simulink model "DDCU_wxt_v02_forA"  (R2014a)
settings: Solver=FixedStepDiscrete  StartTime=0.0  StopTime=50  FixedStep=0.0005  RelTol=1e-3
InitFcn:
  | Veh_Par_wxt
values from neighbouring files (symbols this model uses):
  ag_thr = 0.4*g    (= 3.924)    [Veh_Par_wxt.m]
  B = 2.25    [Veh_Par_wxt.m]
  bra_pre_em = 12    [Veh_Par_wxt.m]
  bra_pre_gz2 = 12/3    (= 4)    [Veh_Par_wxt.m]
  bra_pre_gz34 = 12/3    (= 4)    [Veh_Par_wxt.m]
  bra_pre_yd = 12/2    (= 6)    [Veh_Par_wxt.m]
  brakepre_dem_data = [0 1 2 3 4 5 6 7 8 9 10 11 12]    [Veh_Par_wxt.m]
  brakeTrq_dem_data = [0 218.198 436.396 654.594 872.792 1090.99 1309.188 1527.386 1745.584 1963.782 2181.98 2400.178 2618.376]    [Veh_Par_wxt.m]
  bratrq_max = 4*2618.376    (= 10473.504)    [Veh_Par_wxt.m]
  eff_tran = 0.75    [Veh_Par_wxt.m]
  G = Mass*g    (= 36297)    [Veh_Par_wxt.m]
  kd1 = 1    [Veh_Par_wxt.m]
  kd2 = 1    [Veh_Par_wxt.m]
  kd3 = 1    [Veh_Par_wxt.m]
  ki1 = 1    [Veh_Par_wxt.m]
  ki2 = 1    [Veh_Par_wxt.m]
  ki3 = 1    [Veh_Par_wxt.m]
  kp1 = 1    [Veh_Par_wxt.m]
  kp2 = 1    [Veh_Par_wxt.m]
  kp3 = 1    [Veh_Par_wxt.m]
  L = 3.12    [Veh_Par_wxt.m]
  Radius = 0.20    (= 0.2)    [Veh_Par_wxt.m]
  s_opt_yi_add = 0.05    [Veh_Par_wxt.m]
  s_opt_zhuan_add = 0.05    [Veh_Par_wxt.m]
  spd_map_mot = [0 100 200 300 360 400 500 600 700 800 900]*tras_ratio    [Veh_Par_wxt.m]
  speed_thr_park = 5/3.6/Radius*30/pi    (= 66.3145596216)    [Veh_Par_wxt.m]
  trq_map_mot = [1200 1200 1200 1200 1200 1080 864 720 617 540 480]/tras_ratio    [Veh_Par_wxt.m]
  v_thr1_b = 5    [Veh_Par_wxt.m]
  v_thr2_b = 20    [Veh_Par_wxt.m]
  v_thr_park = 5    [Veh_Par_wxt.m]
undefined symbols (not defined in the file or in its folder): DiscIntNeverNeededParam
libraries: simulink x201, ec5744lib x19
(part 2 of 9)

== matlab function DDCU_wxt_v02_forA/MainControl/mode_control/center_steer/center_steer/容错控制/MATLAB Function ==
  data: trq_dem_l input; trq_dem_lf output; trq_dem_r input; trqlim_lf input; trqlim_lr input; trqlim_rf input; trqlim_rr input; guzhang_lf input; guzhang_lr input; guzhang_rf input; guzhang_rr input; trq_dem_lr output; trq_dem_rf output; trq_dem_rr output; bra_pre_l output; bra_pre_r output; bra_pre_yd input
function [trq_dem_lf,trq_dem_lr,trq_dem_rf,trq_dem_rr,bra_pre_l,bra_pre_r] = fcn(trq_dem_l,trq_dem_r,trqlim_lf,trqlim_lr,trqlim_rf,trqlim_rr,guzhang_lf,guzhang_lr,guzhang_rf,guzhang_rr,bra_pre_yd)
%#codegen
if guzhang_lf==0 && guzhang_lr==0 && guzhang_rf==0 && guzhang_rr==0    %0电机故障,平均分配
    trq_dem_lf=trq_dem_l/2;
    trq_dem_lr=trq_dem_l/2;
    trq_dem_rf=trq_dem_r/2;
    trq_dem_rr=trq_dem_r/2;
    bra_pre_l=0;
    bra_pre_r=0;
elseif  guzhang_lf==1 && guzhang_lr==0 && guzhang_rf==0 && guzhang_rr==0  %1电机故障，同侧电机进行力矩转移,跟行车不同，对侧不降扭。
    trq_dem_lf=0;
    trq_dem_lr=min(trq_dem_l,trqlim_lr);
    trq_dem_rf=trq_dem_r/2;
    trq_dem_rr=trq_dem_r/2;
    bra_pre_l=0;
    bra_pre_r=0;
elseif  guzhang_lf==0 && guzhang_lr==1 && guzhang_rf==0 && guzhang_rr==0
    trq_dem_lf=min(trq_dem_l,trqlim_lf);
    trq_dem_lr=0;
    trq_dem_rf=trq_dem_r/2;
    trq_dem_rr=trq_dem_r/2;
    bra_pre_l=0;
    bra_pre_r=0;
elseif  guzhang_lf==0 && guzhang_lr==0 && guzhang_rf==1 && guzhang_rr==0
    trq_dem_rf=0;
    trq_dem_rr=min(trq_dem_r,trqlim_rr);
    trq_dem_lf=trq_dem_l/2;
    trq_dem_lr=trq_dem_l/2;
    bra_pre_l=0;
    bra_pre_r=0;
elseif  guzhang_lf==0 && guzhang_lr==0 && guzhang_rf==0 && guzhang_rr==1
    trq_dem_rf=min(trq_dem_r,trqlim_rf);
    trq_dem_rr=0;
    trq_dem_lf=trq_dem_l/2;
    trq_dem_lr=trq_dem_l/2;
    bra_pre_l=0;
    bra_pre_r=0;
elseif  guzhang_lf==1 && guzhang_lr==1 && guzhang_rf==0 && guzhang_rr==0  %2电机故障，左侧双电机故障，左侧履带施加制动，改为原地转向
    trq_dem_lf=0;
    trq_dem_lr=0;
    trq_dem_rf=trq_dem_r/2;
    trq_dem_rr=trq_dem_r/2;
    bra_pre_l=bra_pre_yd;
    bra_pre_r=0;
elseif  guzhang_lf==0 && guzhang_lr==0 && guzhang_rf==1 && guzhang_rr==1  %右侧双电机故障
    trq_dem_lf=trq_dem_l/2;
    trq_dem_lr=trq_dem_l/2;
    trq_dem_rf=0;
    trq_dem_rr=0;
    bra_pre_l=0;
    bra_pre_r=bra_pre_yd;
    
elseif  guzhang_lf==1 && guzhang_lr==0 && guzhang_rf==1 && guzhang_rr==0 %2电机故障，对侧双电机故障,有4种情况,前两电机故障
    trq_dem_lf=0;
    trq_dem_rf=0;
    trq_dem_lr=min(trq_dem_l,trqlim_lr);
    trq_dem_rr=min(trq_dem_r,trqlim_rr);
    bra_pre_l=0;
    bra_pre_r=0;
elseif  guzhang_lf==0 && guzhang_lr==1 && guzhang_rf==0 && guzhang_rr==0 %后两电机故障
    trq_dem_lr=0;
    trq_dem_rr=0;
    trq_dem_lf=min(trq_dem_l,trqlim_lf);
    trq_dem_rf=min(trq_dem_r,trqlim_rf);
    bra_pre_l=0;
    bra_pre_r=0;
elseif  guzhang_lf==0 && guzhang_lr==1 && guzhang_rf==0 && guzhang_rr==0 %左前电机和右后电机故障
    trq_dem_lf=0;
    trq_dem_rr=0;
    trq_dem_lr=min(trq_dem_l,trqlim_lr);
    trq_dem_rf=min(trq_dem_r,trqlim_rf);
    bra_pre_l=0;
    bra_pre_r=0;
elseif  guzhang_lf==0 && guzhang_lr==1 && guzhang_rf==0 && guzhang_rr==0 %左后电机和右前电机故障
    trq_dem_lr=0;
    trq_dem_rf=0;
    trq_dem_lf=min(trq_dem_l,trqlim_lf);
    trq_dem_rr=min(trq_dem_r,trqlim_rr);
    bra_pre_l=0;
    bra_pre_r=0;
elseif guzhang_lf==1 && guzhang_lr==1 && guzhang_rf==1 && guzhang_rr==0   % 三电机故障
    trq_dem_lf=0;
    trq_dem_lr=0;
    trq_dem_rf=0;
    trq_dem_rr=min(trq_dem_r,trqlim_rr);
    bra_pre_l=bra_pre_yd;
    bra_pre_r=0;
elseif guzhang_lf==1 && guzhang_lr==1 && guzhang_rf==0 && guzhang_rr==1
    trq_dem_lf=0;
    trq_dem_lr=0;
    trq_dem_rf=min(trq_dem_r,trqlim_rf);
    trq_dem_rr=0;
    bra_pre_l=bra_pre_yd;
    bra_pre_r=0;
elseif guzhang_lf==1 && guzhang_lr==0 && guzhang_rf==1 && guzhang_rr==1
    trq_dem_lf=0;
    trq_dem_lr=min(trq_dem_l,trqlim_lr);
    trq_dem_rf=0;
    trq_dem_rr=0;
    bra_pre_l=0;
    bra_pre_r=bra_pre_yd;
elseif guzhang_lf==0 && guzhang_lr==1 && guzhang_rf==1 && guzhang_rr==1
    trq_dem_lf=min(trq_dem_l,trqlim_lf);
    trq_dem_lr=0;
    trq_dem_rf=0;
    trq_dem_rr=0;
    bra_pre_l=0;
    bra_pre_r=bra_pre_yd;
else
    %     guzhang_lf==1 && guzhang_lr==1 && guzhang_rf==1 && guzhang_rr==1 %四电机故障
    trq_dem_lf=0;
    trq_dem_lr=0;
    trq_dem_rf=0;
    trq_dem_rr=0;
    bra_pre_l=0;
    bra_pre_r=0;
end
end

== system DDCU_wxt_v02_forA/OutputSignalProcess/VCU_MCU2_replace ==
  M4SpeedSet_in : Inport
  M3SpeedSet_in : Inport  Port=2
  MCU2HeartBeat_in : Inport  Port=3
  M4SpeedLimit_in : Inport  Port=4
  M4Mode_in : Inport  Port=5
  M4Enable_in : Inport  Port=6
  M4Drive_in : Inport  Port=7
  M3SpeedLimit_in : Inport  Port=8
  M3Mode_in : Inport  Port=9
  M3Enable_in : Inport  Port=10
  M3Drive_in : Inport  Port=11
  Conv{1..8} (8 alike) : DataTypeConversion
  M3Drive : Subsystem
  M3Enable : Subsystem
  M3Mode : Subsystem
  M3SpeedLimit : Subsystem
  M3SpeedSet : Subsystem
  M4Drive : Subsystem
  M4Enable : Subsystem
  M4Mode : Subsystem
  M4SpeedLimit : Subsystem
  M4SpeedSet : Subsystem
  MCU2HeartBeat : Subsystem
  VCU_MCU2_replace_DLC : Constant  Value=8  OutDataTypeStr=uint8
  VCU_MCU2_replace_DLC_Out : Terminator
  VCU_MCU2_replace_ID : Constant  Value=2348937234  OutDataTypeStr=single
  VCU_MCU2_replace_ID_Out : Terminator
  VCU_MCU2_replace_mux : Mux  Inputs=8
  or{1..8} (8 alike) : simulink/Logic and Bit Operations/Bitwise Operator  logicop=OR  UseBitMask=off  NumInputPorts=11  BitMask=bin2dec('11011001')  BitMaskRealWorld=Stored Integer
  output : Outport
  wires:
  VCU_MCU2_replace_mux/1 -> output/1
  M4SpeedSet/1(output1) -> or1/1
  M4SpeedSet/2(output2) -> or2/1
  M4SpeedSet/3(output3) -> or3/1
  M4SpeedSet/4(output4) -> or4/1
  M4SpeedSet/5(output5) -> or5/1
  M4SpeedSet/6(output6) -> or6/1
  M4SpeedSet/7(output7) -> or7/1
  M4SpeedSet/8(output8) -> or8/1
  M3SpeedSet/1(output1) -> or1/2
  M3SpeedSet/2(output2) -> or2/2
  M3SpeedSet/3(output3) -> or3/2
  M3SpeedSet/4(output4) -> or4/2
  M3SpeedSet/5(output5) -> or5/2
  M3SpeedSet/6(output6) -> or6/2
  M3SpeedSet/7(output7) -> or7/2
  M3SpeedSet/8(output8) -> or8/2
  MCU2HeartBeat/1(output1) -> or1/3
  MCU2HeartBeat/2(output2) -> or2/3
  MCU2HeartBeat/3(output3) -> or3/3
  MCU2HeartBeat/4(output4) -> or4/3
  MCU2HeartBeat/5(output5) -> or5/3
  MCU2HeartBeat/6(output6) -> or6/3
  MCU2HeartBeat/7(output7) -> or7/3
  MCU2HeartBeat/8(output8) -> or8/3
  M4SpeedLimit/1(output1) -> or1/4
  M4SpeedLimit/2(output2) -> or2/4
  M4SpeedLimit/3(output3) -> or3/4
  M4SpeedLimit/4(output4) -> or4/4
  M4SpeedLimit/5(output5) -> or5/4
  M4SpeedLimit/6(output6) -> or6/4
  M4SpeedLimit/7(output7) -> or7/4
  M4SpeedLimit/8(output8) -> or8/4
  M4Mode/1(output1) -> or1/5
  M4Mode/2(output2) -> or2/5
  M4Mode/3(output3) -> or3/5
  M4Mode/4(output4) -> or4/5
  M4Mode/5(output5) -> or5/5
  M4Mode/6(output6) -> or6/5
  M4Mode/7(output7) -> or7/5
  M4Mode/8(output8) -> or8/5
  M4Enable/1(output1) -> or1/6
  M4Enable/2(output2) -> or2/6
  M4Enable/3(output3) -> or3/6
  M4Enable/4(output4) -> or4/6
  M4Enable/5(output5) -> or5/6
  M4Enable/6(output6) -> or6/6
  M4Enable/7(output7) -> or7/6
  M4Enable/8(output8) -> or8/6
  M4Drive/1(output1) -> or1/7
  M4Drive/2(output2) -> or2/7
  M4Drive/3(output3) -> or3/7
  M4Drive/4(output4) -> or4/7
  M4Drive/5(output5) -> or5/7
  M4Drive/6(output6) -> or6/7
  M4Drive/7(output7) -> or7/7
  M4Drive/8(output8) -> or8/7
  M3SpeedLimit/1(output1) -> or1/8
  M3SpeedLimit/2(output2) -> or2/8
  M3SpeedLimit/3(output3) -> or3/8
  M3SpeedLimit/4(output4) -> or4/8
  M3SpeedLimit/5(output5) -> or5/8
  M3SpeedLimit/6(output6) -> or6/8
  M3SpeedLimit/7(output7) -> or7/8
  M3SpeedLimit/8(output8) -> or8/8
  M3Mode/1(output1) -> or1/9
  M3Mode/2(output2) -> or2/9
  M3Mode/3(output3) -> or3/9
  M3Mode/4(output4) -> or4/9
  M3Mode/5(output5) -> or5/9
  M3Mode/6(output6) -> or6/9
  M3Mode/7(output7) -> or7/9
  M3Mode/8(output8) -> or8/9
  M3Enable/1(output1) -> or1/10
  M3Enable/2(output2) -> or2/10
  M3Enable/3(output3) -> or3/10
  M3Enable/4(output4) -> or4/10
  M3Enable/5(output5) -> or5/10
  M3Enable/6(output6) -> or6/10
  M3Enable/7(output7) -> or7/10
  M3Enable/8(output8) -> or8/10
  M3Drive/1(output1) -> or1/11
  M3Drive/2(output2) -> or2/11
  M3Drive/3(output3) -> or3/11
  M3Drive/4(output4) -> or4/11
  M3Drive/5(output5) -> or5/11
  M3Drive/6(output6) -> or6/11
  M3Drive/7(output7) -> or7/11
  M3Drive/8(output8) -> or8/11
  or1/1 -> Conv1/1
  Conv1/1 -> VCU_MCU2_replace_mux/1
  or2/1 -> Conv2/1
  Conv2/1 -> VCU_MCU2_replace_mux/2
  or3/1 -> Conv3/1
  Conv3/1 -> VCU_MCU2_replace_mux/3
  or4/1 -> Conv4/1
  Conv4/1 -> VCU_MCU2_replace_mux/4
  or5/1 -> Conv5/1
  Conv5/1 -> VCU_MCU2_replace_mux/5
  or6/1 -> Conv6/1
  Conv6/1 -> VCU_MCU2_replace_mux/6
  or7/1 -> Conv7/1
  Conv7/1 -> VCU_MCU2_replace_mux/7
  or8/1 -> Conv8/1
  Conv8/1 -> VCU_MCU2_replace_mux/8
  VCU_MCU2_replace_ID/1 -> VCU_MCU2_replace_ID_Out/1
  VCU_MCU2_replace_DLC/1 -> VCU_MCU2_replace_DLC_Out/1
  M4SpeedSet_in/1 -> M4SpeedSet/1(M4SpeedSet)
  M3SpeedSet_in/1 -> M3SpeedSet/1(M3SpeedSet)
  MCU2HeartBeat_in/1 -> MCU2HeartBeat/1(MCU2HeartBeat)
  M4SpeedLimit_in/1 -> M4SpeedLimit/1(M4SpeedLimit)
  M4Mode_in/1 -> M4Mode/1(M4Mode)
  M4Enable_in/1 -> M4Enable/1(M4Enable)
  M4Drive_in/1 -> M4Drive/1(M4Drive)
  M3SpeedLimit_in/1 -> M3SpeedLimit/1(M3SpeedLimit)
  M3Mode_in/1 -> M3Mode/1(M3Mode)
  M3Enable_in/1 -> M3Enable/1(M3Enable)
  M3Drive_in/1 -> M3Drive/1(M3Drive)

== system DDCU_wxt_v02_forA/OutputSignalProcess/VCU_Park ==
  ParkEnable_in : Inport
  Conv{1..8} (8 alike) : DataTypeConversion
  ParkEnable : Subsystem
  VCU_Park_DLC : Constant  Value=8  OutDataTypeStr=uint8
  VCU_Park_DLC_Out : Terminator
  VCU_Park_ID : Constant  Value=2281988666  OutDataTypeStr=single
  VCU_Park_ID_Out : Terminator
  VCU_Park_mux : Mux  Inputs=8
  or{1..8} (8 alike) : simulink/Logic and Bit Operations/Bitwise Operator  logicop=OR  UseBitMask=off  BitMask=bin2dec('11011001')  BitMaskRealWorld=Stored Integer
  output : Outport
  wires:
  VCU_Park_mux/1 -> output/1
  ParkEnable/1(output1) -> or1/1
  ParkEnable/2(output2) -> or2/1
  ParkEnable/3(output3) -> or3/1
  ParkEnable/4(output4) -> or4/1
  ParkEnable/5(output5) -> or5/1
  ParkEnable/6(output6) -> or6/1
  ParkEnable/7(output7) -> or7/1
  ParkEnable/8(output8) -> or8/1
  or1/1 -> Conv1/1
  Conv1/1 -> VCU_Park_mux/1
  or2/1 -> Conv2/1
  Conv2/1 -> VCU_Park_mux/2
  or3/1 -> Conv3/1
  Conv3/1 -> VCU_Park_mux/3
  or4/1 -> Conv4/1
  Conv4/1 -> VCU_Park_mux/4
  or5/1 -> Conv5/1
  Conv5/1 -> VCU_Park_mux/5
  or6/1 -> Conv6/1
  Conv6/1 -> VCU_Park_mux/6
  or7/1 -> Conv7/1
  Conv7/1 -> VCU_Park_mux/7
  or8/1 -> Conv8/1
  Conv8/1 -> VCU_Park_mux/8
  VCU_Park_ID/1 -> VCU_Park_ID_Out/1
  VCU_Park_DLC/1 -> VCU_Park_DLC_Out/1
  ParkEnable_in/1 -> ParkEnable/1(ParkEnable)

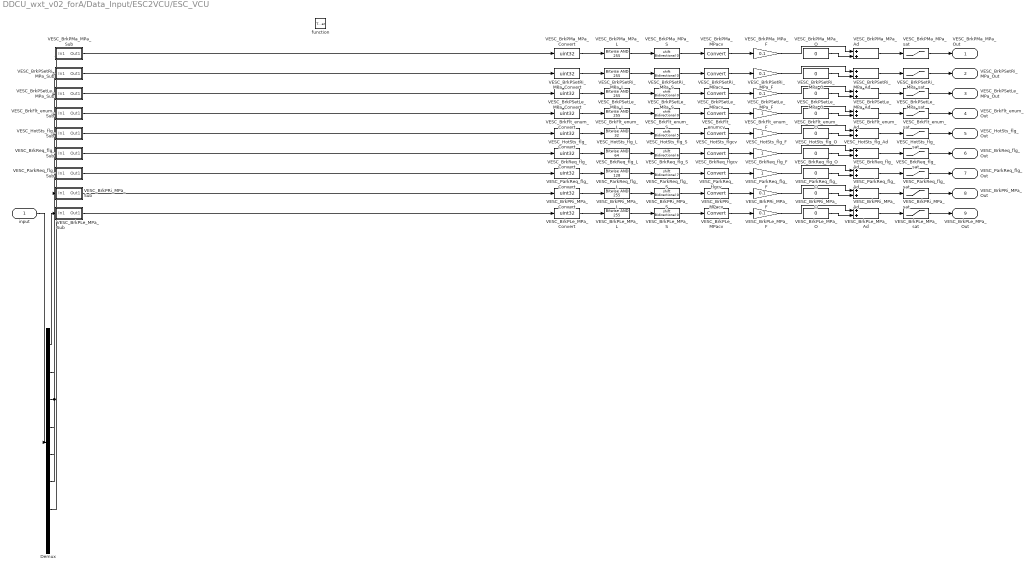
== system DDCU_wxt_v02_forA/Data_Input/ESC2VCU/ESC_VCU ==
  input : Inport
  function : TriggerPort  TriggerType=function-call
  Demux : Demux  Outputs=8
  VESC_BrkFlt_enum_Ad : Sum
  VESC_BrkFlt_enum_Convert : DataTypeConversion  OutDataTypeStr=uint32
  VESC_BrkFlt_enum_F : Gain
  VESC_BrkFlt_enum_L : simulink/Logic and Bit Operations/Bitwise Operator  logicop=AND  UseBitMask=on  BitMask=255  BitMaskRealWorld=Stored Integer
  VESC_BrkFlt_enum_O : Constant  Value=0  OutDataTypeStr=single
  VESC_BrkFlt_enum_S : ArithShift
  VESC_BrkFlt_enum_Sub : Subsystem
  VESC_BrkFlt_enum_sat : Saturate  UpperLimit=255  LowerLimit=0
  VESC_BrkFlt_enumcv : DataTypeConversion
  VESC_BrkPLe_MPa_Ad : Sum
  VESC_BrkPLe_MPa_Convert : DataTypeConversion  OutDataTypeStr=uint32
  VESC_BrkPLe_MPa_F : Gain  Gain=0.1
  VESC_BrkPLe_MPa_L : simulink/Logic and Bit Operations/Bitwise Operator  logicop=AND  UseBitMask=on  BitMask=255  BitMaskRealWorld=Stored Integer
  VESC_BrkPLe_MPa_O : Constant  Value=0  OutDataTypeStr=single
  VESC_BrkPLe_MPa_S : ArithShift
  VESC_BrkPLe_MPa_Sub : Subsystem
  VESC_BrkPLe_MPa_sat : Saturate  UpperLimit=25.5  LowerLimit=0
  VESC_BrkPLe_MPacv : DataTypeConversion
  VESC_BrkPMa_MPa_Ad : Sum
  VESC_BrkPMa_MPa_Convert : DataTypeConversion  OutDataTypeStr=uint32
  VESC_BrkPMa_MPa_F : Gain  Gain=0.1
  VESC_BrkPMa_MPa_L : simulink/Logic and Bit Operations/Bitwise Operator  logicop=AND  UseBitMask=on  BitMask=255  BitMaskRealWorld=Stored Integer
  VESC_BrkPMa_MPa_O : Constant  Value=0  OutDataTypeStr=single
  VESC_BrkPMa_MPa_S : ArithShift
  VESC_BrkPMa_MPa_Sub : Subsystem
  VESC_BrkPMa_MPa_sat : Saturate  UpperLimit=25.5  LowerLimit=0
  VESC_BrkPMa_MPacv : DataTypeConversion
  VESC_BrkPRi_MPa_Ad : Sum
  VESC_BrkPRi_MPa_Convert : DataTypeConversion  OutDataTypeStr=uint32
  VESC_BrkPRi_MPa_F : Gain  Gain=0.1
  VESC_BrkPRi_MPa_L : simulink/Logic and Bit Operations/Bitwise Operator  logicop=AND  UseBitMask=on  BitMask=255  BitMaskRealWorld=Stored Integer
  VESC_BrkPRi_MPa_O : Constant  Value=0  OutDataTypeStr=single
  VESC_BrkPRi_MPa_S : ArithShift
  VESC_BrkPRi_MPa_Sub : Subsystem
  VESC_BrkPRi_MPa_sat : Saturate  UpperLimit=25.5  LowerLimit=0
  VESC_BrkPRi_MPacv : DataTypeConversion
  VESC_BrkPSetLe_MPa_Ad : Sum
  VESC_BrkPSetLe_MPa_Convert : DataTypeConversion  OutDataTypeStr=uint32
  VESC_BrkPSetLe_MPa_F : Gain  Gain=0.1
  VESC_BrkPSetLe_MPa_L : simulink/Logic and Bit Operations/Bitwise Operator  logicop=AND  UseBitMask=on  BitMask=255  BitMaskRealWorld=Stored Integer
  VESC_BrkPSetLe_MPa_O : Constant  Value=0  OutDataTypeStr=single
  VESC_BrkPSetLe_MPa_S : ArithShift
  VESC_BrkPSetLe_MPa_Sub : Subsystem
  VESC_BrkPSetLe_MPa_sat : Saturate  UpperLimit=25.5  LowerLimit=0
  VESC_BrkPSetLe_MPacv : DataTypeConversion
  VESC_BrkPSetRi_MPa_Ad : Sum
  VESC_BrkPSetRi_MPa_Convert : DataTypeConversion  OutDataTypeStr=uint32
  VESC_BrkPSetRi_MPa_F : Gain  Gain=0.1
  VESC_BrkPSetRi_MPa_L : simulink/Logic and Bit Operations/Bitwise Operator  logicop=AND  UseBitMask=on  BitMask=255  BitMaskRealWorld=Stored Integer
  VESC_BrkPSetRi_MPa_O : Constant  Value=0  OutDataTypeStr=single
  VESC_BrkPSetRi_MPa_S : ArithShift
  VESC_BrkPSetRi_MPa_Sub : Subsystem
  VESC_BrkPSetRi_MPa_sat : Saturate  UpperLimit=25.5  LowerLimit=0
  VESC_BrkPSetRi_MPacv : DataTypeConversion
  VESC_BrkReq_flg_Ad : Sum
  VESC_BrkReq_flg_Convert : DataTypeConversion  OutDataTypeStr=uint32
  VESC_BrkReq_flg_F : Gain
  VESC_BrkReq_flg_L : simulink/Logic and Bit Operations/Bitwise Operator  logicop=AND  UseBitMask=on  BitMask=64  BitMaskRealWorld=Stored Integer
  VESC_BrkReq_flg_O : Constant  Value=0  OutDataTypeStr=single
  VESC_BrkReq_flg_S : ArithShift  BitShiftNumber=6
  VESC_BrkReq_flg_Sub : Subsystem
  VESC_BrkReq_flg_sat : Saturate  UpperLimit=1  LowerLimit=0
  VESC_BrkReq_flgcv : DataTypeConversion
  VESC_HotSts_flg_Ad : Sum
  VESC_HotSts_flg_Convert : DataTypeConversion  OutDataTypeStr=uint32
  VESC_HotSts_flg_F : Gain
  VESC_HotSts_flg_L : simulink/Logic and Bit Operations/Bitwise Operator  logicop=AND  UseBitMask=on  BitMask=32  BitMaskRealWorld=Stored Integer
  VESC_HotSts_flg_O : Constant  Value=0  OutDataTypeStr=single
  VESC_HotSts_flg_S : ArithShift  BitShiftNumber=5
  VESC_HotSts_flg_Sub : Subsystem
  VESC_HotSts_flg_sat : Saturate  UpperLimit=1  LowerLimit=0
  VESC_HotSts_flgcv : DataTypeConversion
  VESC_ParkReq_flg_Ad : Sum
  VESC_ParkReq_flg_Convert : DataTypeConversion  OutDataTypeStr=uint32
  VESC_ParkReq_flg_F : Gain
  VESC_ParkReq_flg_L : simulink/Logic and Bit Operations/Bitwise Operator  logicop=AND  UseBitMask=on  BitMask=128  BitMaskRealWorld=Stored Integer
  VESC_ParkReq_flg_O : Constant  Value=0  OutDataTypeStr=single
  VESC_ParkReq_flg_S : ArithShift  BitShiftNumber=7
  VESC_ParkReq_flg_Sub : Subsystem
  VESC_ParkReq_flg_sat : Saturate  UpperLimit=1  LowerLimit=0
  VESC_ParkReq_flgcv : DataTypeConversion
  VESC_BrkPMa_MPa_Out : Outport
  VESC_BrkPSetRi_MPa_Out : Outport  Port=2
  VESC_BrkPSetLe_MPa_Out : Outport  Port=3
  VESC_BrkFlt_enum_Out : Outport  Port=4
  VESC_HotSts_flg_Out : Outport  Port=5
  VESC_BrkReq_flg_Out : Outport  Port=6
  VESC_ParkReq_flg_Out : Outport  Port=7
  VESC_BrkPRi_MPa_Out : Outport  Port=8
  VESC_BrkPLe_MPa_Out : Outport  Port=9
  wires:
  VESC_BrkPMa_MPa_F/1 -> VESC_BrkPMa_MPa_Ad/1
  VESC_BrkPMa_MPa_O/1 -> VESC_BrkPMa_MPa_Ad/2
  VESC_BrkPMa_MPa_Ad/1 -> VESC_BrkPMa_MPa_sat/1
  VESC_BrkPMa_MPa_sat/1 -> VESC_BrkPMa_MPa_Out/1
  Demux/7 -> VESC_BrkPMa_MPa_Sub/1(In1)
  VESC_BrkPMa_MPa_Sub/1(Out1) -> VESC_BrkPMa_MPa_Convert/1
  VESC_BrkPMa_MPa_Convert/1 -> VESC_BrkPMa_MPa_L/1
  VESC_BrkPMa_MPa_L/1 -> VESC_BrkPMa_MPa_S/1
  VESC_BrkPMa_MPa_S/1 -> VESC_BrkPMa_MPacv/1
  VESC_BrkPMa_MPacv/1 -> VESC_BrkPMa_MPa_F/1
  VESC_BrkPSetRi_MPa_F/1 -> VESC_BrkPSetRi_MPa_Ad/1
  VESC_BrkPSetRi_MPa_O/1 -> VESC_BrkPSetRi_MPa_Ad/2
  VESC_BrkPSetRi_MPa_Ad/1 -> VESC_BrkPSetRi_MPa_sat/1
  VESC_BrkPSetRi_MPa_sat/1 -> VESC_BrkPSetRi_MPa_Out/1
  Demux/6 -> VESC_BrkPSetRi_MPa_Sub/1(In1)
  VESC_BrkPSetRi_MPa_Sub/1(Out1) -> VESC_BrkPSetRi_MPa_Convert/1
  VESC_BrkPSetRi_MPa_Convert/1 -> VESC_BrkPSetRi_MPa_L/1
  VESC_BrkPSetRi_MPa_L/1 -> VESC_BrkPSetRi_MPa_S/1
  VESC_BrkPSetRi_MPa_S/1 -> VESC_BrkPSetRi_MPacv/1
  VESC_BrkPSetRi_MPacv/1 -> VESC_BrkPSetRi_MPa_F/1
  VESC_BrkPSetLe_MPa_F/1 -> VESC_BrkPSetLe_MPa_Ad/1
  VESC_BrkPSetLe_MPa_O/1 -> VESC_BrkPSetLe_MPa_Ad/2
  VESC_BrkPSetLe_MPa_Ad/1 -> VESC_BrkPSetLe_MPa_sat/1
  VESC_BrkPSetLe_MPa_sat/1 -> VESC_BrkPSetLe_MPa_Out/1
  Demux/5 -> VESC_BrkPSetLe_MPa_Sub/1(In1)
  VESC_BrkPSetLe_MPa_Sub/1(Out1) -> VESC_BrkPSetLe_MPa_Convert/1
  VESC_BrkPSetLe_MPa_Convert/1 -> VESC_BrkPSetLe_MPa_L/1
  VESC_BrkPSetLe_MPa_L/1 -> VESC_BrkPSetLe_MPa_S/1
  VESC_BrkPSetLe_MPa_S/1 -> VESC_BrkPSetLe_MPacv/1
  VESC_BrkPSetLe_MPacv/1 -> VESC_BrkPSetLe_MPa_F/1
  VESC_BrkFlt_enum_F/1 -> VESC_BrkFlt_enum_Ad/1
  VESC_BrkFlt_enum_O/1 -> VESC_BrkFlt_enum_Ad/2
  VESC_BrkFlt_enum_Ad/1 -> VESC_BrkFlt_enum_sat/1
  VESC_BrkFlt_enum_sat/1 -> VESC_BrkFlt_enum_Out/1
  Demux/4 -> VESC_BrkFlt_enum_Sub/1(In1)
  VESC_BrkFlt_enum_Sub/1(Out1) -> VESC_BrkFlt_enum_Convert/1
  VESC_BrkFlt_enum_Convert/1 -> VESC_BrkFlt_enum_L/1
  VESC_BrkFlt_enum_L/1 -> VESC_BrkFlt_enum_S/1
  VESC_BrkFlt_enum_S/1 -> VESC_BrkFlt_enumcv/1
  VESC_BrkFlt_enumcv/1 -> VESC_BrkFlt_enum_F/1
  VESC_HotSts_flg_F/1 -> VESC_HotSts_flg_Ad/1
  VESC_HotSts_flg_O/1 -> VESC_HotSts_flg_Ad/2
  VESC_HotSts_flg_Ad/1 -> VESC_HotSts_flg_sat/1
  VESC_HotSts_flg_sat/1 -> VESC_HotSts_flg_Out/1
  Demux/3 -> VESC_BrkReq_flg_Sub/1(In1), VESC_ParkReq_flg_Sub/1(In1), VESC_HotSts_flg_Sub/1(In1)
  VESC_HotSts_flg_Sub/1(Out1) -> VESC_HotSts_flg_Convert/1
  VESC_HotSts_flg_Convert/1 -> VESC_HotSts_flg_L/1
  VESC_HotSts_flg_L/1 -> VESC_HotSts_flg_S/1
  VESC_HotSts_flg_S/1 -> VESC_HotSts_flgcv/1
  VESC_HotSts_flgcv/1 -> VESC_HotSts_flg_F/1
  VESC_BrkReq_flg_F/1 -> VESC_BrkReq_flg_Ad/1
  VESC_BrkReq_flg_O/1 -> VESC_BrkReq_flg_Ad/2
  VESC_BrkReq_flg_Ad/1 -> VESC_BrkReq_flg_sat/1
  VESC_BrkReq_flg_sat/1 -> VESC_BrkReq_flg_Out/1
  VESC_BrkReq_flg_Sub/1(Out1) -> VESC_BrkReq_flg_Convert/1
  VESC_BrkReq_flg_Convert/1 -> VESC_BrkReq_flg_L/1
  VESC_BrkReq_flg_L/1 -> VESC_BrkReq_flg_S/1
  VESC_BrkReq_flg_S/1 -> VESC_BrkReq_flgcv/1
  VESC_BrkReq_flgcv/1 -> VESC_BrkReq_flg_F/1
  VESC_ParkReq_flg_F/1 -> VESC_ParkReq_flg_Ad/1
  VESC_ParkReq_flg_O/1 -> VESC_ParkReq_flg_Ad/2
  VESC_ParkReq_flg_Ad/1 -> VESC_ParkReq_flg_sat/1
  VESC_ParkReq_flg_sat/1 -> VESC_ParkReq_flg_Out/1
  VESC_ParkReq_flg_Sub/1(Out1) -> VESC_ParkReq_flg_Convert/1
  VESC_ParkReq_flg_Convert/1 -> VESC_ParkReq_flg_L/1
  VESC_ParkReq_flg_L/1 -> VESC_ParkReq_flg_S/1
  VESC_ParkReq_flg_S/1 -> VESC_ParkReq_flgcv/1
  VESC_ParkReq_flgcv/1 -> VESC_ParkReq_flg_F/1
  VESC_BrkPRi_MPa_F/1 -> VESC_BrkPRi_MPa_Ad/1
  VESC_BrkPRi_MPa_O/1 -> VESC_BrkPRi_MPa_Ad/2
  VESC_BrkPRi_MPa_Ad/1 -> VESC_BrkPRi_MPa_sat/1
  VESC_BrkPRi_MPa_sat/1 -> VESC_BrkPRi_MPa_Out/1
  Demux/2 -> VESC_BrkPRi_MPa_Sub/1(In1)
  VESC_BrkPRi_MPa_Sub/1(Out1) -> VESC_BrkPRi_MPa_Convert/1
  VESC_BrkPRi_MPa_Convert/1 -> VESC_BrkPRi_MPa_L/1
  VESC_BrkPRi_MPa_L/1 -> VESC_BrkPRi_MPa_S/1
  VESC_BrkPRi_MPa_S/1 -> VESC_BrkPRi_MPacv/1
  VESC_BrkPRi_MPacv/1 -> VESC_BrkPRi_MPa_F/1
  VESC_BrkPLe_MPa_F/1 -> VESC_BrkPLe_MPa_Ad/1
  VESC_BrkPLe_MPa_O/1 -> VESC_BrkPLe_MPa_Ad/2
  VESC_BrkPLe_MPa_Ad/1 -> VESC_BrkPLe_MPa_sat/1
  VESC_BrkPLe_MPa_sat/1 -> VESC_BrkPLe_MPa_Out/1
  Demux/1 -> VESC_BrkPLe_MPa_Sub/1(In1)
  VESC_BrkPLe_MPa_Sub/1(Out1) -> VESC_BrkPLe_MPa_Convert/1
  VESC_BrkPLe_MPa_Convert/1 -> VESC_BrkPLe_MPa_L/1
  VESC_BrkPLe_MPa_L/1 -> VESC_BrkPLe_MPa_S/1
  VESC_BrkPLe_MPa_S/1 -> VESC_BrkPLe_MPacv/1
  VESC_BrkPLe_MPacv/1 -> VESC_BrkPLe_MPa_F/1
  input/1 -> Demux/1

== system DDCU_wxt_v02_forA/Data_Input/ESC2VCU/Park1_VCU ==
  input : Inport
  function : TriggerPort  TriggerType=function-call
  Demux : Demux  Outputs=8
  ParkZiJian_Ad : Sum
  ParkZiJian_Convert : DataTypeConversion  OutDataTypeStr=uint32
  ParkZiJian_F : Gain
  ParkZiJian_L : simulink/Logic and Bit Operations/Bitwise Operator  logicop=AND  UseBitMask=on  BitMask=1  BitMaskRealWorld=Stored Integer
  ParkZiJian_O : Constant  Value=0  OutDataTypeStr=single
  ParkZiJian_S : ArithShift
  ParkZiJian_Sub : Subsystem
  ParkZiJian_sat : Saturate  UpperLimit=1  LowerLimit=0
  ParkZiJiancv : DataTypeConversion
  ParkZiJian_Out : Outport
  wires:
  ParkZiJian_F/1 -> ParkZiJian_Ad/1
  ParkZiJian_O/1 -> ParkZiJian_Ad/2
  ParkZiJian_Ad/1 -> ParkZiJian_sat/1
  ParkZiJian_sat/1 -> ParkZiJian_Out/1
  Demux/2 -> ParkZiJian_Sub/1(In1)
  ParkZiJian_Sub/1(Out1) -> ParkZiJian_Convert/1
  ParkZiJian_Convert/1 -> ParkZiJian_L/1
  ParkZiJian_L/1 -> ParkZiJian_S/1
  ParkZiJian_S/1 -> ParkZiJiancv/1
  ParkZiJiancv/1 -> ParkZiJian_F/1
  input/1 -> Demux/1

== system DDCU_wxt_v02_forA/Data_Input/ESC2VCU/Park2_VCU ==
  input : Inport
  function : TriggerPort  TriggerType=function-call
  Demux : Demux  Outputs=8
  ParkState_Ad : Sum
  ParkState_Convert : DataTypeConversion  OutDataTypeStr=uint32
  ParkState_F : Gain
  ParkState_L : simulink/Logic and Bit Operations/Bitwise Operator  logicop=AND  UseBitMask=on  BitMask=1  BitMaskRealWorld=Stored Integer
  ParkState_O : Constant  Value=0  OutDataTypeStr=single
  ParkState_S : ArithShift
  ParkState_Sub : Subsystem
  ParkState_sat : Saturate  UpperLimit=1  LowerLimit=0
  ParkStatecv : DataTypeConversion
  ParkState_Out : Outport
  wires:
  ParkState_F/1 -> ParkState_Ad/1
  ParkState_O/1 -> ParkState_Ad/2
  ParkState_Ad/1 -> ParkState_sat/1
  ParkState_sat/1 -> ParkState_Out/1
  Demux/2 -> ParkState_Sub/1(In1)
  ParkState_Sub/1(Out1) -> ParkState_Convert/1
  ParkState_Convert/1 -> ParkState_L/1
  ParkState_L/1 -> ParkState_S/1
  ParkState_S/1 -> ParkStatecv/1
  ParkStatecv/1 -> ParkState_F/1
  input/1 -> Demux/1

== system DDCU_wxt_v02_forA/Data_Input/HCU2VCU/HCU1_VCU ==
  input : Inport
  function : TriggerPort  TriggerType=function-call
  Demux : Demux  Outputs=8
  HCUState_Ad : Sum
  HCUState_Convert : DataTypeConversion  OutDataTypeStr=uint32
  HCUState_F : Gain
  HCUState_L : simulink/Logic and Bit Operations/Bitwise Operator  logicop=AND  UseBitMask=on  BitMask=63  BitMaskRealWorld=Stored Integer
  HCUState_O : Constant  Value=0  OutDataTypeStr=single
  HCUState_S : ArithShift
  HCUState_Sub : Subsystem
  HCUState_sat : Saturate  UpperLimit=63  LowerLimit=0
  HCUStatecv : DataTypeConversion
  KeyState_Ad : Sum
  KeyState_Convert : DataTypeConversion  OutDataTypeStr=uint32
  KeyState_F : Gain
  KeyState_L : simulink/Logic and Bit Operations/Bitwise Operator  logicop=AND  UseBitMask=on  BitMask=3  BitMaskRealWorld=Stored Integer
  KeyState_O : Constant  Value=0  OutDataTypeStr=single
  KeyState_S : ArithShift
  KeyState_Sub : Subsystem
  KeyState_sat : Saturate  UpperLimit=3  LowerLimit=0
  KeyStatecv : DataTypeConversion
  VehEnvironment_Ad : Sum
  VehEnvironment_Convert : DataTypeConversion  OutDataTypeStr=uint32
  VehEnvironment_F : Gain
  VehEnvironment_L : simulink/Logic and Bit Operations/Bitwise Operator  logicop=AND  UseBitMask=on  BitMask=12  BitMaskRealWorld=Stored Integer
  VehEnvironment_O : Constant  Value=0  OutDataTypeStr=single
  VehEnvironment_S : ArithShift  BitShiftNumber=2
  VehEnvironment_Sub : Subsystem
  VehEnvironment_sat : Saturate  UpperLimit=3  LowerLimit=0
  VehEnvironmentcv : DataTypeConversion
  VehFault_Ad : Sum
  VehFault_Convert : DataTypeConversion  OutDataTypeStr=uint32
  VehFault_F : Gain
  VehFault_L : simulink/Logic and Bit Operations/Bitwise Operator  logicop=AND  UseBitMask=on  BitMask=192  BitMaskRealWorld=Stored Integer
  VehFault_O : Constant  Value=0  OutDataTypeStr=single
  VehFault_S : ArithShift  BitShiftNumber=6
  VehFault_Sub : Subsystem
  VehFault_sat : Saturate  UpperLimit=3  LowerLimit=0
  VehFaultcv : DataTypeConversion
  VehEnvironment_Out : Outport
  KeyState_Out : Outport  Port=2
  VehFault_Out : Outport  Port=3
  HCUState_Out : Outport  Port=4
  wires:
  VehEnvironment_F/1 -> VehEnvironment_Ad/1
  VehEnvironment_O/1 -> VehEnvironment_Ad/2
  VehEnvironment_Ad/1 -> VehEnvironment_sat/1
  VehEnvironment_sat/1 -> VehEnvironment_Out/1
  Demux/3 -> VehEnvironment_Sub/1(In1), KeyState_Sub/1(In1)
  VehEnvironment_Sub/1(Out1) -> VehEnvironment_Convert/1
  VehEnvironment_Convert/1 -> VehEnvironment_L/1
  VehEnvironment_L/1 -> VehEnvironment_S/1
  VehEnvironment_S/1 -> VehEnvironmentcv/1
  VehEnvironmentcv/1 -> VehEnvironment_F/1
  KeyState_F/1 -> KeyState_Ad/1
  KeyState_O/1 -> KeyState_Ad/2
  KeyState_Ad/1 -> KeyState_sat/1
  KeyState_sat/1 -> KeyState_Out/1
  KeyState_Sub/1(Out1) -> KeyState_Convert/1
  KeyState_Convert/1 -> KeyState_L/1
  KeyState_L/1 -> KeyState_S/1
  KeyState_S/1 -> KeyStatecv/1
  KeyStatecv/1 -> KeyState_F/1
  VehFault_F/1 -> VehFault_Ad/1
  VehFault_O/1 -> VehFault_Ad/2
  VehFault_Ad/1 -> VehFault_sat/1
  VehFault_sat/1 -> VehFault_Out/1
  Demux/2 -> VehFault_Sub/1(In1), HCUState_Sub/1(In1)
  VehFault_Sub/1(Out1) -> VehFault_Convert/1
  VehFault_Convert/1 -> VehFault_L/1
  VehFault_L/1 -> VehFault_S/1
  VehFault_S/1 -> VehFaultcv/1
  VehFaultcv/1 -> VehFault_F/1
  HCUState_F/1 -> HCUState_Ad/1
  HCUState_O/1 -> HCUState_Ad/2
  HCUState_Ad/1 -> HCUState_sat/1
  HCUState_sat/1 -> HCUState_Out/1
  HCUState_Sub/1(Out1) -> HCUState_Convert/1
  HCUState_Convert/1 -> HCUState_L/1
  HCUState_L/1 -> HCUState_S/1
  HCUState_S/1 -> HCUStatecv/1
  HCUStatecv/1 -> HCUState_F/1
  input/1 -> Demux/1

== system DDCU_wxt_v02_forA/Data_Input/HCU2VCU/HCU2_VCU ==
  input : Inport
  function : TriggerPort  TriggerType=function-call
  AccBra_Ad : Sum
  AccBra_Convert : DataTypeConversion  OutDataTypeStr=uint32
  AccBra_F : Gain  Gain=0.5
  AccBra_L : simulink/Logic and Bit Operations/Bitwise Operator  logicop=AND  UseBitMask=on  BitMask=255  BitMaskRealWorld=Stored Integer
  AccBra_O : Constant  Value=0  OutDataTypeStr=single
  AccBra_S : ArithShift
  AccBra_Sub : Subsystem
  AccBra_sat : Saturate  UpperLimit=127.5  LowerLimit=0
  AccBracv : DataTypeConversion
  Demux : Demux  Outputs=8
  Mode1_Ad : Sum
  Mode1_Convert : DataTypeConversion  OutDataTypeStr=uint32
  Mode1_F : Gain
  Mode1_L : simulink/Logic and Bit Operations/Bitwise Operator  logicop=AND  UseBitMask=on  BitMask=15  BitMaskRealWorld=Stored Integer
  Mode1_O : Constant  Value=0  OutDataTypeStr=single
  Mode1_S : ArithShift
  Mode1_Sub : Subsystem
  Mode1_sat : Saturate  UpperLimit=15  LowerLimit=0
  Mode1cv : DataTypeConversion
  Mode2_Ad : Sum
  Mode2_Convert : DataTypeConversion  OutDataTypeStr=uint32
  Mode2_F : Gain
  Mode2_L : simulink/Logic and Bit Operations/Bitwise Operator  logicop=AND  UseBitMask=on  BitMask=240  BitMaskRealWorld=Stored Integer
  Mode2_O : Constant  Value=0  OutDataTypeStr=single
  Mode2_S : ArithShift  BitShiftNumber=4
  Mode2_Sub : Subsystem
  Mode2_sat : Saturate  UpperLimit=15  LowerLimit=0
  Mode2cv : DataTypeConversion
  Turn_Ad : Sum
  Turn_Convert : DataTypeConversion  OutDataTypeStr=uint32
  Turn_F : Gain
  Turn_L : simulink/Logic and Bit Operations/Bitwise Operator  logicop=AND  UseBitMask=on  BitMask=255  BitMaskRealWorld=Stored Integer
  Turn_O : Constant  Value=-125  OutDataTypeStr=single
  Turn_S : ArithShift
  Turn_Sub : Subsystem
  Turn_sat : Saturate  UpperLimit=130  LowerLimit=-125
  Turncv : DataTypeConversion
  Turn_Out : Outport
  AccBra_Out : Outport  Port=2
  Mode2_Out : Outport  Port=3
  Mode1_Out : Outport  Port=4
  wires:
  Turn_F/1 -> Turn_Ad/1
  Turn_O/1 -> Turn_Ad/2
  Turn_Ad/1 -> Turn_sat/1
  Turn_sat/1 -> Turn_Out/1
  Demux/8 -> Turn_Sub/1(In1)
  Turn_Sub/1(Out1) -> Turn_Convert/1
  Turn_Convert/1 -> Turn_L/1
  Turn_L/1 -> Turn_S/1
  Turn_S/1 -> Turncv/1
  Turncv/1 -> Turn_F/1
  AccBra_F/1 -> AccBra_Ad/1
  AccBra_O/1 -> AccBra_Ad/2
  AccBra_Ad/1 -> AccBra_sat/1
  AccBra_sat/1 -> AccBra_Out/1
  Demux/5 -> AccBra_Sub/1(In1)
  AccBra_Sub/1(Out1) -> AccBra_Convert/1
  AccBra_Convert/1 -> AccBra_L/1
  AccBra_L/1 -> AccBra_S/1
  AccBra_S/1 -> AccBracv/1
  AccBracv/1 -> AccBra_F/1
  Mode2_F/1 -> Mode2_Ad/1
  Mode2_O/1 -> Mode2_Ad/2
  Mode2_Ad/1 -> Mode2_sat/1
  Mode2_sat/1 -> Mode2_Out/1
  Demux/2 -> Mode2_Sub/1(In1), Mode1_Sub/1(In1)
  Mode2_Sub/1(Out1) -> Mode2_Convert/1
  Mode2_Convert/1 -> Mode2_L/1
  Mode2_L/1 -> Mode2_S/1
  Mode2_S/1 -> Mode2cv/1
  Mode2cv/1 -> Mode2_F/1
  Mode1_F/1 -> Mode1_Ad/1
  Mode1_O/1 -> Mode1_Ad/2
  Mode1_Ad/1 -> Mode1_sat/1
  Mode1_sat/1 -> Mode1_Out/1
  Mode1_Sub/1(Out1) -> Mode1_Convert/1
  Mode1_Convert/1 -> Mode1_L/1
  Mode1_L/1 -> Mode1_S/1
  Mode1_S/1 -> Mode1cv/1
  Mode1cv/1 -> Mode1_F/1
  input/1 -> Demux/1

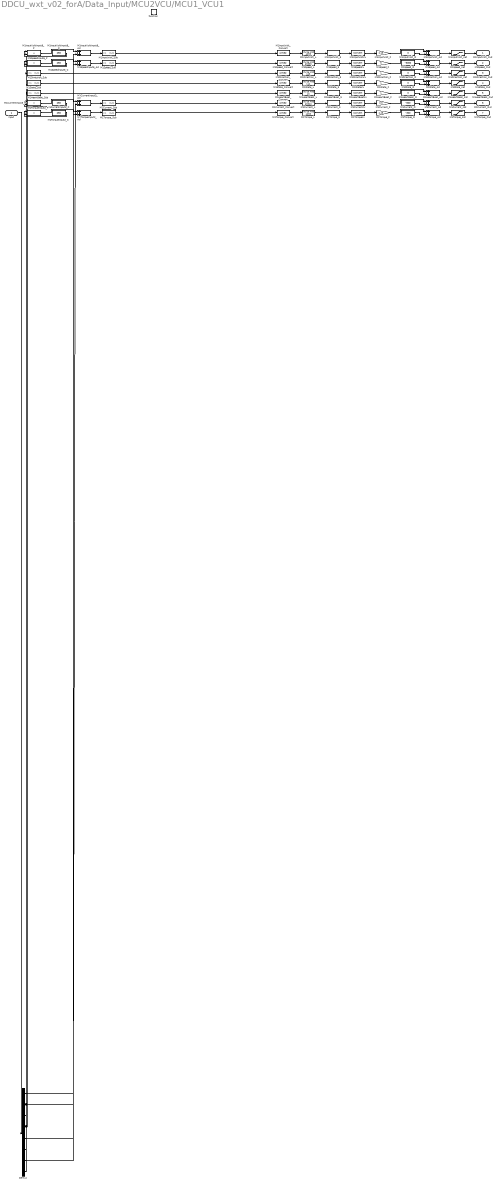
== system DDCU_wxt_v02_forA/Data_Input/MCU2VCU/MCU1_VCU1 ==
  input : Inport
  function : TriggerPort  TriggerType=function-call
  Demux : Demux  Outputs=8
  M1Current_Ad : Sum
  M1Current_Convert : DataTypeConversion  OutDataTypeStr=uint32
  M1Current_F : Gain  Gain=0.5
  M1Current_L : simulink/Logic and Bit Operations/Bitwise Operator  logicop=AND  UseBitMask=on  BitMask=65520  BitMaskRealWorld=Stored Integer
  M1Current_O : Constant  Value=-600  OutDataTypeStr=single
  M1Current_S : ArithShift  BitShiftNumber=4
  M1Current_Sub : Subsystem
  M1Current_sat : Saturate  UpperLimit=1447.5  LowerLimit=-600
  M1Currentcv : DataTypeConversion
  M1Currentinput3_Ad : Sum
  M1Currentinput3_C : Constant  Value=256
  M1Currentinput3_P : Product
  M1Direction_Ad : Sum
  M1Direction_Convert : DataTypeConversion  OutDataTypeStr=uint32
  M1Direction_F : Gain
  M1Direction_L : simulink/Logic and Bit Operations/Bitwise Operator  logicop=AND  UseBitMask=on  BitMask=128  BitMaskRealWorld=Stored Integer
  M1Direction_O : Constant  Value=0  OutDataTypeStr=single
  M1Direction_S : ArithShift  BitShiftNumber=7
  M1Direction_Sub : Subsystem
  M1Direction_sat : Saturate  UpperLimit=1  LowerLimit=0
  M1Directioncv : DataTypeConversion
  M1HeartBeat_Ad : Sum
  M1HeartBeat_Convert : DataTypeConversion  OutDataTypeStr=uint32
  M1HeartBeat_F : Gain
  M1HeartBeat_L : simulink/Logic and Bit Operations/Bitwise Operator  logicop=AND  UseBitMask=on  BitMask=15  BitMaskRealWorld=Stored Integer
  M1HeartBeat_O : Constant  Value=0  OutDataTypeStr=single
  M1HeartBeat_S : ArithShift
  M1HeartBeat_Sub : Subsystem
  M1HeartBeat_sat : Saturate  UpperLimit=15  LowerLimit=0
  M1HeartBeatcv : DataTypeConversion
  M1InputVolt_Ad : Sum
  M1InputVolt_Convert : DataTypeConversion  OutDataTypeStr=uint32
  M1InputVolt_F : Gain  Gain=0.25
  M1InputVolt_L : simulink/Logic and Bit Operations/Bitwise Operator  logicop=AND  UseBitMask=on  BitMask=4095  BitMaskRealWorld=Stored Integer
  M1InputVolt_O : Constant  Value=0  OutDataTypeStr=single
  M1InputVolt_S : ArithShift
  M1InputVolt_Sub : Subsystem
  M1InputVolt_sat : Saturate  UpperLimit=1023.75  LowerLimit=0
  M1InputVoltcv : DataTypeConversion
  M1InputVoltinput8_Ad : Sum
  M1InputVoltinput8_C : Constant  Value=256
  M1InputVoltinput8_P : Product
  M1Speed_Ad : Sum
  M1Speed_Convert : DataTypeConversion  OutDataTypeStr=uint32
  M1Speed_F : Gain  Gain=5
  M1Speed_L : simulink/Logic and Bit Operations/Bitwise Operator  logicop=AND  UseBitMask=on  BitMask=65535  BitMaskRealWorld=Stored Integer
  M1Speed_O : Constant  Value=-5000  OutDataTypeStr=single
  M1Speed_S : ArithShift
  M1Speed_Sub : Subsystem
  M1Speed_sat : Saturate  UpperLimit=322675  LowerLimit=-5000
  M1Speedcv : DataTypeConversion
  M1Speedinput6_Ad : Sum
  M1Speedinput6_C : Constant  Value=256
  M1Speedinput6_P : Product
  M1State_Ad : Sum
  M1State_Convert : DataTypeConversion  OutDataTypeStr=uint32
  M1State_F : Gain
  M1State_L : simulink/Logic and Bit Operations/Bitwise Operator  logicop=AND  UseBitMask=on  BitMask=112  BitMaskRealWorld=Stored Integer
  M1State_O : Constant  Value=0  OutDataTypeStr=single
  M1State_S : ArithShift  BitShiftNumber=4
  M1State_Sub : Subsystem
  M1State_sat : Saturate  UpperLimit=7  LowerLimit=0
  M1Statecv : DataTypeConversion
  M1Torque_Ad : Sum
  M1Torque_Convert : DataTypeConversion  OutDataTypeStr=uint32
  M1Torque_F : Gain  Gain=0.25
  M1Torque_L : simulink/Logic and Bit Operations/Bitwise Operator  logicop=AND  UseBitMask=on  BitMask=4095  BitMaskRealWorld=Stored Integer
  M1Torque_O : Constant  Value=-300  OutDataTypeStr=single
  M1Torque_S : ArithShift
  M1Torque_Sub : Subsystem
  M1Torque_sat : Saturate  UpperLimit=723.75  LowerLimit=-300
  M1Torquecv : DataTypeConversion
  M1Torqueinput2_Ad : Sum
  M1Torqueinput2_C : Constant  Value=256
  M1Torqueinput2_P : Product
  M1InputVolt_Out : Outport
  M1Speed_Out : Outport  Port=2
  M1Direction_Out : Outport  Port=3
  M1State_Out : Outport  Port=4
  M1HeartBeat_Out : Outport  Port=5
  M1Current_Out : Outport  Port=6
  M1Torque_Out : Outport  Port=7
  wires:
  M1InputVolt_F/1 -> M1InputVolt_Ad/1
  M1InputVolt_O/1 -> M1InputVolt_Ad/2
  M1InputVolt_Ad/1 -> M1InputVolt_sat/1
  M1InputVolt_sat/1 -> M1InputVolt_Out/1
  Demux/8 -> M1InputVoltinput8_P/1
  M1InputVoltinput8_C/1 -> M1InputVoltinput8_P/2
  M1InputVoltinput8_P/1 -> M1InputVoltinput8_Ad/1
  Demux/7 -> M1InputVoltinput8_Ad/2
  M1InputVoltinput8_Ad/1 -> M1InputVolt_Sub/1(In1)
  M1InputVolt_Sub/1(Out1) -> M1InputVolt_Convert/1
  M1InputVolt_Convert/1 -> M1InputVolt_L/1
  M1InputVolt_L/1 -> M1InputVolt_S/1
  M1InputVolt_S/1 -> M1InputVoltcv/1
  M1InputVoltcv/1 -> M1InputVolt_F/1
  M1Speed_F/1 -> M1Speed_Ad/1
  M1Speed_O/1 -> M1Speed_Ad/2
  M1Speed_Ad/1 -> M1Speed_sat/1
  M1Speed_sat/1 -> M1Speed_Out/1
  Demux/6 -> M1Speedinput6_P/1
  M1Speedinput6_C/1 -> M1Speedinput6_P/2
  M1Speedinput6_P/1 -> M1Speedinput6_Ad/1
  Demux/5 -> M1Speedinput6_Ad/2
  M1Speedinput6_Ad/1 -> M1Speed_Sub/1(In1)
  M1Speed_Sub/1(Out1) -> M1Speed_Convert/1
  M1Speed_Convert/1 -> M1Speed_L/1
  M1Speed_L/1 -> M1Speed_S/1
  M1Speed_S/1 -> M1Speedcv/1
  M1Speedcv/1 -> M1Speed_F/1
  M1Direction_F/1 -> M1Direction_Ad/1
  M1Direction_O/1 -> M1Direction_Ad/2
  M1Direction_Ad/1 -> M1Direction_sat/1
  M1Direction_sat/1 -> M1Direction_Out/1
  Demux/4 -> M1State_Sub/1(In1), M1HeartBeat_Sub/1(In1), M1Direction_Sub/1(In1)
  M1Direction_Sub/1(Out1) -> M1Direction_Convert/1
  M1Direction_Convert/1 -> M1Direction_L/1
  M1Direction_L/1 -> M1Direction_S/1
  M1Direction_S/1 -> M1Directioncv/1
  M1Directioncv/1 -> M1Direction_F/1
  M1State_F/1 -> M1State_Ad/1
  M1State_O/1 -> M1State_Ad/2
  M1State_Ad/1 -> M1State_sat/1
  M1State_sat/1 -> M1State_Out/1
  M1State_Sub/1(Out1) -> M1State_Convert/1
  M1State_Convert/1 -> M1State_L/1
  M1State_L/1 -> M1State_S/1
  M1State_S/1 -> M1Statecv/1
  M1Statecv/1 -> M1State_F/1
  M1HeartBeat_F/1 -> M1HeartBeat_Ad/1
  M1HeartBeat_O/1 -> M1HeartBeat_Ad/2
  M1HeartBeat_Ad/1 -> M1HeartBeat_sat/1
  M1HeartBeat_sat/1 -> M1HeartBeat_Out/1
  M1HeartBeat_Sub/1(Out1) -> M1HeartBeat_Convert/1
  M1HeartBeat_Convert/1 -> M1HeartBeat_L/1
  M1HeartBeat_L/1 -> M1HeartBeat_S/1
  M1HeartBeat_S/1 -> M1HeartBeatcv/1
  M1HeartBeatcv/1 -> M1HeartBeat_F/1
  M1Current_F/1 -> M1Current_Ad/1
  M1Current_O/1 -> M1Current_Ad/2
  M1Current_Ad/1 -> M1Current_sat/1
  M1Current_sat/1 -> M1Current_Out/1
  Demux/3 -> M1Currentinput3_P/1
  M1Currentinput3_C/1 -> M1Currentinput3_P/2
  M1Currentinput3_P/1 -> M1Currentinput3_Ad/1
  Demux/2 -> M1Currentinput3_Ad/2, M1Torqueinput2_P/1
  M1Currentinput3_Ad/1 -> M1Current_Sub/1(In1)
  M1Current_Sub/1(Out1) -> M1Current_Convert/1
  M1Current_Convert/1 -> M1Current_L/1
  M1Current_L/1 -> M1Current_S/1
  M1Current_S/1 -> M1Currentcv/1
  M1Currentcv/1 -> M1Current_F/1
  M1Torque_F/1 -> M1Torque_Ad/1
  M1Torque_O/1 -> M1Torque_Ad/2
  M1Torque_Ad/1 -> M1Torque_sat/1
  M1Torque_sat/1 -> M1Torque_Out/1
  M1Torqueinput2_C/1 -> M1Torqueinput2_P/2
  M1Torqueinput2_P/1 -> M1Torqueinput2_Ad/1
  Demux/1 -> M1Torqueinput2_Ad/2
  M1Torqueinput2_Ad/1 -> M1Torque_Sub/1(In1)
  M1Torque_Sub/1(Out1) -> M1Torque_Convert/1
  M1Torque_Convert/1 -> M1Torque_L/1
  M1Torque_L/1 -> M1Torque_S/1
  M1Torque_S/1 -> M1Torquecv/1
  M1Torquecv/1 -> M1Torque_F/1
  input/1 -> Demux/1

== system DDCU_wxt_v02_forA/Data_Input/MCU2VCU/MCU1_VCU2 ==
  input : Inport
  function : TriggerPort  TriggerType=function-call
  Demux : Demux  Outputs=8
  M1FaultCode_Ad : Sum
  M1FaultCode_Convert : DataTypeConversion  OutDataTypeStr=uint32
  M1FaultCode_F : Gain
  M1FaultCode_L : simulink/Logic and Bit Operations/Bitwise Operator  logicop=AND  UseBitMask=on  BitMask=65520  BitMaskRealWorld=Stored Integer
  M1FaultCode_O : Constant  Value=0  OutDataTypeStr=single
  M1FaultCode_S : ArithShift  BitShiftNumber=4
  M1FaultCode_Sub : Subsystem
  M1FaultCode_sat : Saturate  UpperLimit=4095  LowerLimit=0
  M1FaultCodecv : DataTypeConversion
  M1FaultCodeinput8_Ad : Sum
  M1FaultCodeinput8_C : Constant  Value=256
  M1FaultCodeinput8_P : Product
  M1FaultGrade_Ad : Sum
  M1FaultGrade_Convert : DataTypeConversion  OutDataTypeStr=uint32
  M1FaultGrade_F : Gain
  M1FaultGrade_L : simulink/Logic and Bit Operations/Bitwise Operator  logicop=AND  UseBitMask=on  BitMask=15  BitMaskRealWorld=Stored Integer
  M1FaultGrade_O : Constant  Value=0  OutDataTypeStr=single
  M1FaultGrade_S : ArithShift
  M1FaultGrade_Sub : Subsystem
  M1FaultGrade_sat : Saturate  UpperLimit=15  LowerLimit=0
  M1FaultGradecv : DataTypeConversion
  M1IGBTTemp_Ad : Sum
  M1IGBTTemp_Convert : DataTypeConversion  OutDataTypeStr=uint32
  M1IGBTTemp_F : Gain
  M1IGBTTemp_L : simulink/Logic and Bit Operations/Bitwise Operator  logicop=AND  UseBitMask=on  BitMask=255  BitMaskRealWorld=Stored Integer
  M1IGBTTemp_O : Constant  Value=-50  OutDataTypeStr=single
  M1IGBTTemp_S : ArithShift
  M1IGBTTemp_Sub : Subsystem
  M1IGBTTemp_sat : Saturate  UpperLimit=205  LowerLimit=-50
  M1IGBTTempcv : DataTypeConversion
  M1Temp_Ad : Sum
  M1Temp_Convert : DataTypeConversion  OutDataTypeStr=uint32
  M1Temp_F : Gain
  M1Temp_L : simulink/Logic and Bit Operations/Bitwise Operator  logicop=AND  UseBitMask=on  BitMask=255  BitMaskRealWorld=Stored Integer
  M1Temp_O : Constant  Value=-50  OutDataTypeStr=single
  M1Temp_S : ArithShift
  M1Temp_Sub : Subsystem
  M1Temp_sat : Saturate  UpperLimit=205  LowerLimit=-50
  M1Tempcv : DataTypeConversion
  M1TqLimit_Ad : Sum
  M1TqLimit_Convert : DataTypeConversion  OutDataTypeStr=uint32
  M1TqLimit_F : Gain  Gain=0.125
  M1TqLimit_L : simulink/Logic and Bit Operations/Bitwise Operator  logicop=AND  UseBitMask=on  BitMask=65535  BitMaskRealWorld=Stored Integer
  M1TqLimit_O : Constant  Value=0  OutDataTypeStr=single
  M1TqLimit_S : ArithShift
  M1TqLimit_Sub : Subsystem
  M1TqLimit_sat : Saturate  UpperLimit=8191.875  LowerLimit=0
  M1TqLimitcv : DataTypeConversion
  M1TqLimitinput6_Ad : Sum
  M1TqLimitinput6_C : Constant  Value=256
  M1TqLimitinput6_P : Product
  M1FaultGrade_Out : Outport
  M1FaultCode_Out : Outport  Port=2
  M1TqLimit_Out : Outport  Port=3
  M1IGBTTemp_Out : Outport  Port=4
  M1Temp_Out : Outport  Port=5
  wires:
  M1FaultGrade_F/1 -> M1FaultGrade_Ad/1
  M1FaultGrade_O/1 -> M1FaultGrade_Ad/2
  M1FaultGrade_Ad/1 -> M1FaultGrade_sat/1
  M1FaultGrade_sat/1 -> M1FaultGrade_Out/1
  Demux/7 -> M1FaultGrade_Sub/1(In1), M1FaultCodeinput8_Ad/2
  M1FaultGrade_Sub/1(Out1) -> M1FaultGrade_Convert/1
  M1FaultGrade_Convert/1 -> M1FaultGrade_L/1
  M1FaultGrade_L/1 -> M1FaultGrade_S/1
  M1FaultGrade_S/1 -> M1FaultGradecv/1
  M1FaultGradecv/1 -> M1FaultGrade_F/1
  M1FaultCode_F/1 -> M1FaultCode_Ad/1
  M1FaultCode_O/1 -> M1FaultCode_Ad/2
  M1FaultCode_Ad/1 -> M1FaultCode_sat/1
  M1FaultCode_sat/1 -> M1FaultCode_Out/1
  Demux/8 -> M1FaultCodeinput8_P/1
  M1FaultCodeinput8_C/1 -> M1FaultCodeinput8_P/2
  M1FaultCodeinput8_P/1 -> M1FaultCodeinput8_Ad/1
  M1FaultCodeinput8_Ad/1 -> M1FaultCode_Sub/1(In1)
  M1FaultCode_Sub/1(Out1) -> M1FaultCode_Convert/1
  M1FaultCode_Convert/1 -> M1FaultCode_L/1
  M1FaultCode_L/1 -> M1FaultCode_S/1
  M1FaultCode_S/1 -> M1FaultCodecv/1
  M1FaultCodecv/1 -> M1FaultCode_F/1
  M1TqLimit_F/1 -> M1TqLimit_Ad/1
  M1TqLimit_O/1 -> M1TqLimit_Ad/2
  M1TqLimit_Ad/1 -> M1TqLimit_sat/1
  M1TqLimit_sat/1 -> M1TqLimit_Out/1
  Demux/6 -> M1TqLimitinput6_P/1
  M1TqLimitinput6_C/1 -> M1TqLimitinput6_P/2
  M1TqLimitinput6_P/1 -> M1TqLimitinput6_Ad/1
  Demux/5 -> M1TqLimitinput6_Ad/2
  M1TqLimitinput6_Ad/1 -> M1TqLimit_Sub/1(In1)
  M1TqLimit_Sub/1(Out1) -> M1TqLimit_Convert/1
  M1TqLimit_Convert/1 -> M1TqLimit_L/1
  M1TqLimit_L/1 -> M1TqLimit_S/1
  M1TqLimit_S/1 -> M1TqLimitcv/1
  M1TqLimitcv/1 -> M1TqLimit_F/1
  M1IGBTTemp_F/1 -> M1IGBTTemp_Ad/1
  M1IGBTTemp_O/1 -> M1IGBTTemp_Ad/2
  M1IGBTTemp_Ad/1 -> M1IGBTTemp_sat/1
  M1IGBTTemp_sat/1 -> M1IGBTTemp_Out/1
  Demux/2 -> M1IGBTTemp_Sub/1(In1)
  M1IGBTTemp_Sub/1(Out1) -> M1IGBTTemp_Convert/1
  M1IGBTTemp_Convert/1 -> M1IGBTTemp_L/1
  M1IGBTTemp_L/1 -> M1IGBTTemp_S/1
  M1IGBTTemp_S/1 -> M1IGBTTempcv/1
  M1IGBTTempcv/1 -> M1IGBTTemp_F/1
  M1Temp_F/1 -> M1Temp_Ad/1
  M1Temp_O/1 -> M1Temp_Ad/2
  M1Temp_Ad/1 -> M1Temp_sat/1
  M1Temp_sat/1 -> M1Temp_Out/1
  Demux/1 -> M1Temp_Sub/1(In1)
  M1Temp_Sub/1(Out1) -> M1Temp_Convert/1
  M1Temp_Convert/1 -> M1Temp_L/1
  M1Temp_L/1 -> M1Temp_S/1
  M1Temp_S/1 -> M1Tempcv/1
  M1Tempcv/1 -> M1Temp_F/1
  input/1 -> Demux/1
